simulink model "Trajectory"  (R2019a)
settings: Solver=VariableStepAuto  StartTime=0.0  StopTime=5  RelTol=1e-3
libraries: simulink x1
settings Model: Creator=DongDung  LastModifiedBy=DongDung

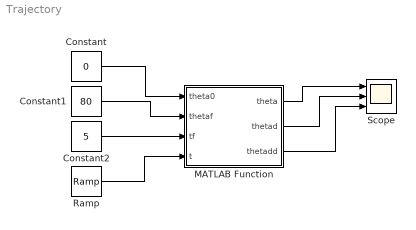
== system Trajectory ==
  Constant : Constant  Value=0
  Constant1 : Constant  Value=80
  Constant2 : Constant  Value=5
  MATLAB Function : MATLAB Function  TreatAsAtomicUnit=on
  Ramp : simulink/Sources/Ramp  slope=1  start=0  InitialOutput=5
  Scope : Scope  NumInputPorts=3
  wires:
  Constant/1 -> MATLAB Function/1(theta0)
  Constant1/1 -> MATLAB Function/2(thetaf)
  MATLAB Function/1(theta) -> Scope/1
  MATLAB Function/2(thetad) -> Scope/2
  MATLAB Function/3(thetadd) -> Scope/3
  Constant2/1 -> MATLAB Function/3(tf)
  Ramp/1 -> MATLAB Function/4(t)

== matlab function Trajectory/MATLAB Function ==
  data: theta0 input; theta output; thetaf input; tf input; thetad output; thetadd output; t input
function [theta, thetad, thetadd] = fcn(theta0,thetaf,tf,t)
a3 = -2*(thetaf-theta0)/tf^3;
a2 =  3*(thetaf-theta0)/tf^2;
theta = a3*t.^3 + a2*t.^2 + theta0;
thetad = 3*a3*t.^2 + 2*a2*t;
thetadd=6*a3*t + 2*a2;
